simulink model "chap9_5sim"  (R2015a)
settings: Solver=ode45  StartTime=0.0  StopTime=30  RelTol=1e-3
settings Model: Creator=zhr  LastModifiedBy=IT

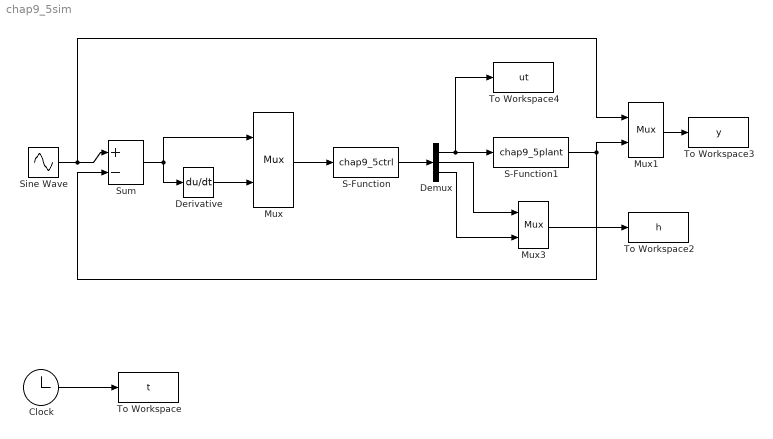
== system chap9_5sim ==
  Clock : Clock
  Demux : Demux  Outputs=3
  Derivative : Derivative
  Mux : Mux  Inputs=2
  Mux1 : Mux  Inputs=2
  Mux3 : Mux  Inputs=2
  S-Function : S-Function  FunctionName=chap9_5ctrl
  S-Function1 : S-Function  FunctionName=chap9_5plant
  Sine Wave : Sin  Amplitude=0.1  SampleTime=0
  Sum : Sum  Inputs=+-
  To Workspace : ToWorkspace  VariableName=t  SampleTime=-1
  To Workspace2 : ToWorkspace  VariableName=h  SampleTime=-1
  To Workspace3 : ToWorkspace  VariableName=y  SampleTime=-1
  To Workspace4 : ToWorkspace  VariableName=ut  SampleTime=-1
  wires:
  Clock/1 -> To Workspace/1
  Sine Wave/1 -> Mux1/1, Sum/1
  Sum/1 -> Derivative/1, Mux/1
  Derivative/1 -> Mux/2
  Mux/1 -> S-Function/1
  S-Function/1 -> Demux/1
  Demux/1 -> To Workspace4/1, S-Function1/1
  S-Function1/1 -> Mux1/2, Sum/2
  Mux1/1 -> To Workspace3/1
  Mux3/1 -> To Workspace2/1
  Demux/2 -> Mux3/1
  Demux/3 -> Mux3/2
